simulink model "basic_pid_torque_postSPEA"  (R2015a)
settings: Solver=ode45  StartTime=0.0  StopTime=10.0  RelTol=1e-3
values from neighbouring files (symbols this model uses):
  k_p = 1    [parameters.m]
  k_s = i    [multi_pass.m]    (also in parameters.m = 124)
  pid_torque_Kd = 0    [parameters.m]
  pid_torque_Ki = 0    [parameters.m]
  pid_torque_Kp = 0    [parameters.m]
  tau_max = 5    [parameters.m]
undefined symbols (not defined in the file or in its folder): pid
libraries: simulink x1
settings Model: Creator=preston  LastModifiedBy=Nathan

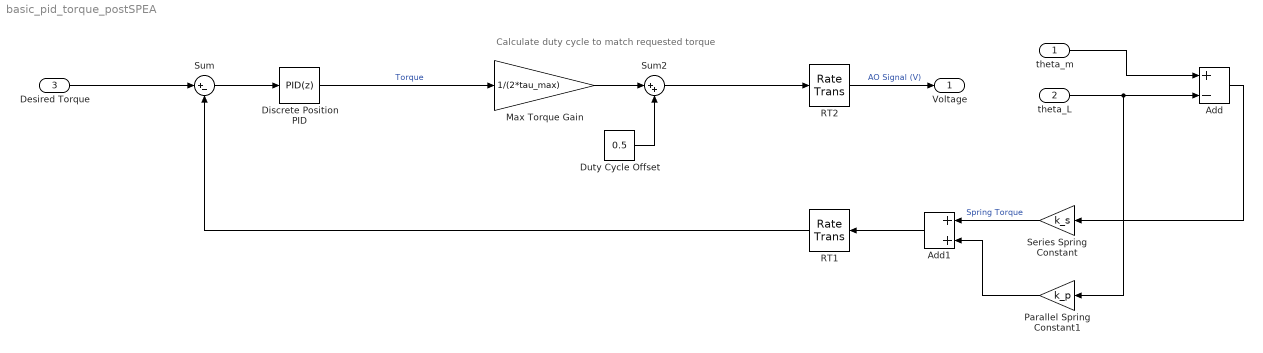
== system basic_pid_torque_postSPEA ==
  note: Calculate duty cycle to match requested torque
  theta_m : Inport
  theta_L : Inport  Port=2
  Desired Torque : Inport  Port=3
  Add : Sum  Inputs=+-
  Add1 : Sum
  Discrete Position PID : simulink/Continuous/PID Controller  Controller=PID  TimeDomain=Discrete-time  SampleTime=-1  IntegratorMethod=Backward Euler  FilterMethod=Forward Euler  Form=Parallel  UseFilter=off  ControllerParametersSource=internal  P=pid_torque_Kp  I=pid_torque_Ki  D=pid_torque_Kd  N=pid.N  InitialConditionSource=internal  InitialConditionForIntegrator=0  InitialConditionForFilter=0  ExternalReset=none  LimitOutput=on  UpperSaturationLimit=tau_max  LowerSaturationLimit=-tau_max  LinearizeAsGain=off  AntiWindupMode=none  Kb=1  TrackingMode=off  Kt=1  PParamMin=[]  PParamMax=[]  IParamMin=[]  IParamMax=[]  DParamMin=[]  DParamMax=[]  NParamMin=[]  NParamMax=[]  KbParamMin=[]  KbParamMax=[]  KtParamMin=[]  KtParamMax=[]  POutMin=[]  POutMax=[]  IOutMin=[]  IOutMax=[]  DOutMin=[]  DOutMax=[]  NOutMin=[]  NOutMax=[]  KbOutMin=[]  KbOutMax=[]  KtOutMin=[]  KtOutMax=[]  IntegratorOutMin=[]  IntegratorOutMax=[]  FilterOutMin=[]  FilterOutMax=[]  SumOutMin=[]  SumOutMax=[]  SumI1OutMin=[]  SumI1OutMax=[]  SumI2OutMin=[]  SumI2OutMax=[]  SumI3OutMin=[]  SumI3OutMax=[]  SumDOutMin=[]  SumDOutMax=[]  SaturationOutMin=[]  SaturationOutMax=[]  IntegratorContinuousStateAttributes=''  IntegratorStateMustResolveToSignalObject=off  IntegratorRTWStateStorageClass=Auto  FilterContinuousStateAttributes=''  FilterStateMustResolveToSignalObject=off  FilterRTWStateStorageClass=Auto  DifferentiatorICPrevScaledInput=0  DifferentiatorOutMin=[]  DifferentiatorOutMax=[]
  Duty Cycle Offset : Constant  Value=0.5
  Max Torque Gain : Gain  Gain=1/(2*tau_max)
  Parallel Spring Constant1 : Gain  Gain=k_p
  RT1 : RateTransition  OutPortSampleTime=T_sample_control
  RT2 : RateTransition
  Series Spring Constant : Gain  Gain=k_s
  Sum : Sum  Inputs=|+-
  Sum2 : Sum  Inputs=|++
  Voltage : Outport
  wires:
  RT2/1 -> Voltage/1  "AO Signal (V)"
  Sum/1 -> Discrete Position PID/1
  Add/1 -> Series Spring Constant/1
  RT1/1 -> Sum/2
  theta_m/1 -> Add/1
  theta_L/1 -> Parallel Spring Constant1/1, Add/2
  Desired Torque/1 -> Sum/1
  Series Spring Constant/1 -> Add1/1  "Spring Torque"
  Parallel Spring Constant1/1 -> Add1/2
  Add1/1 -> RT1/1
  Discrete Position PID/1 -> Max Torque Gain/1  "Torque"
  Max Torque Gain/1 -> Sum2/1
  Sum2/1 -> RT2/1
  Duty Cycle Offset/1 -> Sum2/2
